simulink model "moving_avg_filter"  (R2017b)
settings: Solver=VariableStepAuto  StartTime=0.0  StopTime=43.418  RelTol=1e-3
libraries: dsparch4 x1, dspstat3 x1
settings Model: Creator=jadevarelle  LastModifiedBy=Zach
settings CodeAppCC: StateflowObjectComments=on

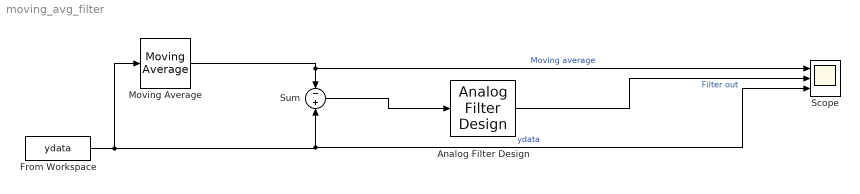
== system moving_avg_filter ==
  Analog Filter Design : dsparch4/Analog Filter Design  method=Butterworth  filttype=Bandpass  N=8  Wlo=0.5  Whi=5  Rp=2  Rs=40
  From Workspace : FromWorkspace  VariableName=ydata  SampleTime=0.02  OutputAfterFinalValue=Setting to zero
  Moving Average : dspstat3/Moving Average  Method=Exponential weighting  SpecifyWindowLength=on  WindowLength=300  ForgettingFactor=1  SimulateUsing=Code generation
  Scope : Scope  NumInputPorts=3
  Sum : Sum  Inputs=-|+
  wires:
  From Workspace/1 -> Scope/3, Sum/2, Moving Average/1  "ydata"
  Moving Average/1 -> Sum/1, Scope/1  "Moving average"
  Sum/1 -> Analog Filter Design/1
  Analog Filter Design/1 -> Scope/2  "Filter out"
